simulink model "test_frictionalPumpMotor"  (R2013a)
settings: Solver=ode45  StartTime=0.0  StopTime=10.0  RelTol=1e-3
libraries: fl_lib x9, nesl_utility x4, usask_hyd_lib x1
settings Model: Creator=tkw954  LastModifiedBy=tkw954
settings SimscapeCC: SimscapeLogType=all  SimscapeLogLimitData=off

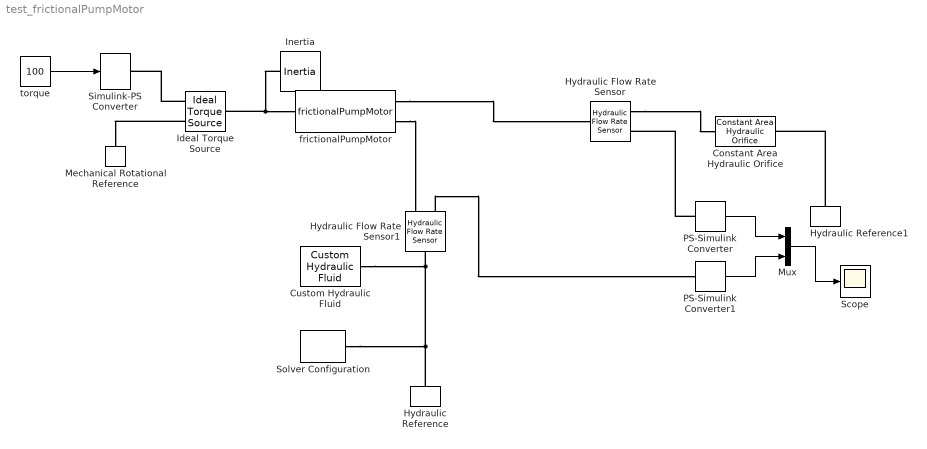
== system test_frictionalPumpMotor ==
  Constant Area Hydraulic Orifice : fl_lib/Hydraulic/Hydraulic Elements/Constant Area Hydraulic Orifice  area=1e-4 m^2  C_d=0.7  Re_cr=12  C_d_lam=0.0408  D_h=0.0113 m  q_Log=off  p_Log=off  LocalVarNames=|q|p  LocalVarDescs=|q|p  LocalVarLogging=[0 0]
  Custom Hydraulic Fluid : fl_lib/Hydraulic/Hydraulic Utilities/Custom Hydraulic Fluid  density=850 kg/m^3  viscosity_kin=18e-6 m^2/s  bulk=0.8e9 Pa  alpha=0.005  LocalVarLogging=[]
  Hydraulic Flow Rate Sensor : fl_lib/Hydraulic/Hydraulic Sensors/Hydraulic Flow Rate Sensor  q_Log=off  p_Log=off  LocalVarNames=|q|p  LocalVarDescs=|q|p  LocalVarLogging=[0 0]
  Hydraulic Flow Rate Sensor1 : fl_lib/Hydraulic/Hydraulic Sensors/Hydraulic Flow Rate Sensor  q_Log=off  p_Log=off  LocalVarNames=|q|p  LocalVarDescs=|q|p  LocalVarLogging=[0 0]
  Hydraulic Reference : fl_lib/Hydraulic/Hydraulic Elements/Hydraulic Reference  q_Log=off  LocalVarNames=|q  LocalVarDescs=|q  LocalVarLogging=0
  Hydraulic Reference1 : fl_lib/Hydraulic/Hydraulic Elements/Hydraulic Reference  q_Log=off  LocalVarNames=|q  LocalVarDescs=|q  LocalVarLogging=0
  Ideal Torque Source : fl_lib/Mechanical/Mechanical Sources/Ideal Torque Source  w_Log=off  t_Log=off  LocalVarNames=|w|t  LocalVarDescs=|w|t  LocalVarLogging=[0 0]
  Inertia : fl_lib/Mechanical/Rotational Elements/Inertia  inertia=0.5 kg*m^2  initial_velocity=0 rad/s  t_Log=off  LocalVarNames=|t  LocalVarDescs=|t  LocalVarLogging=0
  Mechanical Rotational Reference : fl_lib/Mechanical/Rotational Elements/Mechanical Rotational Reference  t_Log=off  LocalVarNames=|t  LocalVarDescs=|t  LocalVarLogging=0
  Mux : Mux  Inputs=2
  PS-Simulink Converter : nesl_utility/PS-Simulink Converter  PhysicalDomain=network_engine_domain  SubClassName=ps_output  LeftPortType=input  RightPortType=output  PseudoPeriodic=off  Frequencies=[]  Unit=1  AffineConversion=off
  PS-Simulink Converter1 : nesl_utility/PS-Simulink Converter  PhysicalDomain=network_engine_domain  SubClassName=ps_output  LeftPortType=input  RightPortType=output  PseudoPeriodic=off  Frequencies=[]  Unit=1  AffineConversion=off
  Scope : Scope
  Simulink-PS Converter : nesl_utility/Simulink-PS Converter  PhysicalDomain=network_engine_domain  SubClassName=ps_input  LeftPortType=input  RightPortType=output  PseudoPeriodic=off  Frequencies=[]  NoiseDistribution=none  NoiseParameters=[]  Unit=N*m  AffineConversion=off  InputFiltering=off  SimscapeFilterOrder=1  InputFilterTimeConstant=0.001  UdotUserProvided=1
  Solver Configuration : nesl_utility/Solver Configuration  PhysicalDomain=network_engine_domain  SubClassName=solver  LeftPortType=input  RightPortType=generic  Accelerate=off  Tones=[]  Harmonics=[]  SimulateNoise=off  Profile=off  UseLocalSampling=off  EnableSwitchedLinearOptims=on  FrequencyDomain=off  UseCCode=off  UseNewInitialization=off  DoDC=off  ResidualTolerance=1e-09  UseLocalSolver=off  LocalSolverChoice=NE_BACKWARD_EULER_ADVANCER  LocalSolverSampleTime=0.001  DoFixedCost=off  MaxNonlinIter=3  MaxModeIter=2  LinearAlgebra=Sparse  DelaysMemoryBudget=1024
  frictionalPumpMotor : usask_hyd_lib/frictionalPumpMotor  D=200e-6  T_br=25  T_c=20  B_f=0.001  trans_coef=10  V_thresh=1e-4
  torque : Constant  Value=100
  wires:
  torque/1 -> Simulink-PS Converter/1
  PS-Simulink Converter/1 -> Mux/1
  PS-Simulink Converter1/1 -> Mux/2
  Mux/1 -> Scope/1
  connections:
  Inertia/LConn1 -- frictionalPumpMotor/LConn1 -- Ideal Torque Source/LConn1
  Ideal Torque Source/RConn2 -- Mechanical Rotational Reference/LConn1
  Ideal Torque Source/RConn1 -- Simulink-PS Converter/RConn1
  Hydraulic Reference/LConn1 -- Solver Configuration/RConn1 -- Custom Hydraulic Fluid/RConn1 -- Hydraulic Flow Rate Sensor1/LConn1
  Hydraulic Reference1/LConn1 -- Constant Area Hydraulic Orifice/RConn1
  frictionalPumpMotor/RConn2 -- Hydraulic Flow Rate Sensor/LConn1
  Hydraulic Flow Rate Sensor/RConn2 -- Constant Area Hydraulic Orifice/LConn1
  PS-Simulink Converter/LConn1 -- Hydraulic Flow Rate Sensor/RConn1
  Hydraulic Flow Rate Sensor1/RConn1 -- PS-Simulink Converter1/LConn1
  frictionalPumpMotor/RConn1 -- Hydraulic Flow Rate Sensor1/RConn2
